simulink model "case4"  (R2024b)
settings: Solver=FixedStepAuto  StartTime=0  StopTime=1  FixedStep=1e-7  RelTol=1e-3
values from neighbouring files (symbols this model uses):
  SG_D_1_D = 0.01056    [IEEE9_case_parameters.m]    (also in case1_parameters.m; case2_parameters.m; case3_parameters.m; case4_parameters.m)
  SG_D_1_EnableSaturation = 0    [IEEE9_case_parameters.m]    (also in case1_parameters.m; case2_parameters.m; case3_parameters.m; case4_parameters.m)
  SG_D_1_f0 = 60    [IEEE9_case_parameters.m]    (also in case1_parameters.m; case2_parameters.m; case3_parameters.m; case4_parameters.m)
  SG_D_1_H = 7.5    [IEEE9_case_parameters.m]    (also in case1_parameters.m; case2_parameters.m; case3_parameters.m; case4_parameters.m)
  SG_D_1_K_A = 20    [IEEE9_case_parameters.m]    (also in case1_parameters.m; case2_parameters.m; case3_parameters.m; case4_parameters.m)
  SG_D_1_K_E = 1.000000e+1    (= 10)    [IEEE9_case_parameters.m]    (also in case1_parameters.m; case2_parameters.m; case3_parameters.m; case4_parameters.m)
  SG_D_1_K_F = 2.363    [IEEE9_case_parameters.m]    (also in case1_parameters.m; case2_parameters.m; case3_parameters.m; case4_parameters.m)
  SG_D_1_K_s = 0.5    [IEEE9_case_parameters.m]    (also in case1_parameters.m = 5; case2_parameters.m = 5; case3_parameters.m = 5; case4_parameters.m = 5)
  SG_D_1_R_a = 0.001088    [IEEE9_case_parameters.m]    (also in case1_parameters.m; case2_parameters.m; case3_parameters.m; case4_parameters.m)
  SG_D_1_S_A = 1    [IEEE9_case_parameters.m]    (also in case1_parameters.m; case2_parameters.m; case3_parameters.m; case4_parameters.m)
  SG_D_1_S_B = 0.103    [IEEE9_case_parameters.m]    (also in case1_parameters.m; case2_parameters.m; case3_parameters.m; case4_parameters.m)
  SG_D_1_S_N = 10.659857    [IEEE9_case_parameters.m]    (also in case1_parameters.m; case2_parameters.m; case3_parameters.m; case4_parameters.m)
  SG_D_1_SpeedPara = 200    [IEEE9_case_parameters.m]    (also in case1_parameters.m; case2_parameters.m; case3_parameters.m; case4_parameters.m)
  SG_D_1_T_0 = 0.720173    [IEEE9_case_parameters.m]    (also in case1_parameters.m = 0.755522; case2_parameters.m = 0.808931; case3_parameters.m = 0.869402; case4_parameters.m = 0.729316)
  SG_D_1_T_1 = 0.3    [IEEE9_case_parameters.m]    (also in case1_parameters.m; case2_parameters.m; case3_parameters.m; case4_parameters.m)
  SG_D_1_T_2 = 0.05    [IEEE9_case_parameters.m]    (also in case1_parameters.m; case2_parameters.m; case3_parameters.m; case4_parameters.m)
  SG_D_1_T_3 = 0.02    [IEEE9_case_parameters.m]    (also in case1_parameters.m; case2_parameters.m; case3_parameters.m; case4_parameters.m)
  SG_D_1_T_4 = 0.005    [IEEE9_case_parameters.m]    (also in case1_parameters.m; case2_parameters.m; case3_parameters.m; case4_parameters.m)
  SG_D_1_T_A = 0.02    [IEEE9_case_parameters.m]    (also in case1_parameters.m; case2_parameters.m; case3_parameters.m; case4_parameters.m)
  SG_D_1_T_dd = 8.000000e+0    (= 8)    [IEEE9_case_parameters.m]    (also in case1_parameters.m; case2_parameters.m; case3_parameters.m; case4_parameters.m)
  SG_D_1_T_ddd = 0.04    [IEEE9_case_parameters.m]    (also in case1_parameters.m; case2_parameters.m; case3_parameters.m; case4_parameters.m)
  SG_D_1_T_E = 0.314    [IEEE9_case_parameters.m]    (also in case1_parameters.m; case2_parameters.m; case3_parameters.m; case4_parameters.m)
  SG_D_1_T_F = 0.35    [IEEE9_case_parameters.m]    (also in case1_parameters.m; case2_parameters.m; case3_parameters.m; case4_parameters.m)
  SG_D_1_T_qd = 0.8    [IEEE9_case_parameters.m]    (also in case1_parameters.m; case2_parameters.m; case3_parameters.m; case4_parameters.m)
  SG_D_1_T_qdd = 0.02    [IEEE9_case_parameters.m]    (also in case1_parameters.m; case2_parameters.m; case3_parameters.m; case4_parameters.m)
  SG_D_1_T_speed = 0.1    [IEEE9_case_parameters.m]    (also in case1_parameters.m = 200; case2_parameters.m = 200; case3_parameters.m = 200; case4_parameters.m = 200)
  SG_D_1_T_w = 0.5    [IEEE9_case_parameters.m]    (also in case1_parameters.m; case2_parameters.m; case3_parameters.m; case4_parameters.m)
  SG_D_1_V_ref = 1.990276    [IEEE9_case_parameters.m]    (also in case1_parameters.m = 2.042296; case2_parameters.m = 2.051388; case3_parameters.m = 2.089584; case4_parameters.m = 2.01845)
  SG_D_1_w_ref = 376.991118    [IEEE9_case_parameters.m]    (also in case1_parameters.m; case2_parameters.m; case3_parameters.m; case4_parameters.m)
  SG_D_1_wb = 6.000000e+1    (= 60)    [IEEE9_case_parameters.m]    (also in case1_parameters.m; case2_parameters.m; case3_parameters.m; case4_parameters.m)
  SG_D_1_x_d = 1.9    [IEEE9_case_parameters.m]    (also in case1_parameters.m; case2_parameters.m; case3_parameters.m; case4_parameters.m)
  SG_D_1_x_dd = 0.302    [IEEE9_case_parameters.m]    (also in case1_parameters.m; case2_parameters.m; case3_parameters.m; case4_parameters.m)
  SG_D_1_x_ddd = 0.204    [IEEE9_case_parameters.m]    (also in case1_parameters.m; case2_parameters.m; case3_parameters.m; case4_parameters.m)
  SG_D_1_x_l = 0.05    [IEEE9_case_parameters.m]    (also in case1_parameters.m; case2_parameters.m; case3_parameters.m; case4_parameters.m)
  SG_D_1_x_q = 1.3    [IEEE9_case_parameters.m]    (also in case1_parameters.m; case2_parameters.m; case3_parameters.m; case4_parameters.m)
  SG_D_1_x_qd = 0.5    [IEEE9_case_parameters.m]    (also in case1_parameters.m; case2_parameters.m; case3_parameters.m; case4_parameters.m)
  SG_D_1_x_qdd = 0.3    [IEEE9_case_parameters.m]    (also in case1_parameters.m; case2_parameters.m; case3_parameters.m; case4_parameters.m)
  SG_D_2_D = 0.02    [IEEE9_case_parameters.m]    (also in case1_parameters.m; case2_parameters.m; case3_parameters.m; case4_parameters.m)
  SG_D_2_EnableSaturation = 0    [IEEE9_case_parameters.m]    (also in case1_parameters.m; case2_parameters.m; case3_parameters.m; case4_parameters.m)
  SG_D_2_f0 = 60    [IEEE9_case_parameters.m]    (also in case1_parameters.m; case2_parameters.m; case3_parameters.m; case4_parameters.m)
  SG_D_2_H = 8.000000e+0    (= 8)    [IEEE9_case_parameters.m]    (also in case1_parameters.m; case2_parameters.m; case3_parameters.m; case4_parameters.m)
  SG_D_2_K_A = 20    [IEEE9_case_parameters.m]    (also in case1_parameters.m; case2_parameters.m; case3_parameters.m; case4_parameters.m)
  SG_D_2_K_E = 1.000000e+1    (= 10)    [IEEE9_case_parameters.m]    (also in case1_parameters.m; case2_parameters.m; case3_parameters.m; case4_parameters.m)
  SG_D_2_K_F = 2.363    [IEEE9_case_parameters.m]    (also in case1_parameters.m; case2_parameters.m; case3_parameters.m; case4_parameters.m)
  SG_D_2_K_s = 0.5    [IEEE9_case_parameters.m]    (also in case1_parameters.m = 4; case2_parameters.m = 4; case3_parameters.m = 4; case4_parameters.m = 4)
  SG_D_2_R_a = 0.001088    [IEEE9_case_parameters.m]    (also in case1_parameters.m; case2_parameters.m; case3_parameters.m; case4_parameters.m)
  SG_D_2_S_A = 1    [IEEE9_case_parameters.m]    (also in case1_parameters.m; case2_parameters.m; case3_parameters.m; case4_parameters.m)
  SG_D_2_S_B = 0.103    [IEEE9_case_parameters.m]    (also in case1_parameters.m; case2_parameters.m; case3_parameters.m; case4_parameters.m)
  SG_D_2_S_N = 10.659857    [IEEE9_case_parameters.m]    (also in case1_parameters.m; case2_parameters.m; case3_parameters.m; case4_parameters.m)
  SG_D_2_SpeedPara = 200    [IEEE9_case_parameters.m]    (also in case1_parameters.m; case2_parameters.m; case3_parameters.m; case4_parameters.m)
  SG_D_2_T_0 = 1.632913    [IEEE9_case_parameters.m]    (also in case1_parameters.m = 1.632925; case2_parameters.m = 1.632915; case3_parameters.m = 1.632914; case4_parameters.m = 1.632927)
  SG_D_2_T_1 = 0.2    [IEEE9_case_parameters.m]    (also in case1_parameters.m; case2_parameters.m; case3_parameters.m; case4_parameters.m)
  SG_D_2_T_2 = 0.05    [IEEE9_case_parameters.m]    (also in case1_parameters.m; case2_parameters.m; case3_parameters.m; case4_parameters.m)
  SG_D_2_T_3 = 0.02    [IEEE9_case_parameters.m]    (also in case1_parameters.m; case2_parameters.m; case3_parameters.m; case4_parameters.m)
  SG_D_2_T_4 = 0.005    [IEEE9_case_parameters.m]    (also in case1_parameters.m; case2_parameters.m; case3_parameters.m; case4_parameters.m)
  SG_D_2_T_A = 0.02    [IEEE9_case_parameters.m]    (also in case1_parameters.m; case2_parameters.m; case3_parameters.m; case4_parameters.m)
  SG_D_2_T_dd = 7.9    [IEEE9_case_parameters.m]    (also in case1_parameters.m; case2_parameters.m; case3_parameters.m; case4_parameters.m)
  SG_D_2_T_ddd = 0.04    [IEEE9_case_parameters.m]    (also in case1_parameters.m; case2_parameters.m; case3_parameters.m; case4_parameters.m)
  SG_D_2_T_E = 0.314    [IEEE9_case_parameters.m]    (also in case1_parameters.m; case2_parameters.m; case3_parameters.m; case4_parameters.m)
  SG_D_2_T_F = 0.35    [IEEE9_case_parameters.m]    (also in case1_parameters.m; case2_parameters.m; case3_parameters.m; case4_parameters.m)
  SG_D_2_T_qd = 0.8    [IEEE9_case_parameters.m]    (also in case1_parameters.m; case2_parameters.m; case3_parameters.m; case4_parameters.m)
  SG_D_2_T_qdd = 0.015    [IEEE9_case_parameters.m]    (also in case1_parameters.m; case2_parameters.m; case3_parameters.m; case4_parameters.m)
  SG_D_2_T_speed = 0.1    [IEEE9_case_parameters.m]    (also in case1_parameters.m = 150; case2_parameters.m = 150; case3_parameters.m = 150; case4_parameters.m = 150)
  SG_D_2_T_w = 0.35    [IEEE9_case_parameters.m]    (also in case1_parameters.m; case2_parameters.m; case3_parameters.m; case4_parameters.m)
  SG_D_2_V_ref = 2.58547    [IEEE9_case_parameters.m]    (also in case1_parameters.m = 2.597896; case2_parameters.m = 2.587136; case3_parameters.m = 2.586042; case4_parameters.m = 2.599679)
  SG_D_2_w_ref = 376.991118    [IEEE9_case_parameters.m]    (also in case1_parameters.m; case2_parameters.m; case3_parameters.m; case4_parameters.m)
  SG_D_2_wb = 6.000000e+1    (= 60)    [IEEE9_case_parameters.m]    (also in case1_parameters.m; case2_parameters.m; case3_parameters.m; case4_parameters.m)
  SG_D_2_x_d = 1.8    [IEEE9_case_parameters.m]    (also in case1_parameters.m; case2_parameters.m; case3_parameters.m; case4_parameters.m)
  SG_D_2_x_dd = 0.302    [IEEE9_case_parameters.m]    (also in case1_parameters.m; case2_parameters.m; case3_parameters.m; case4_parameters.m)
  SG_D_2_x_ddd = 0.204    [IEEE9_case_parameters.m]    (also in case1_parameters.m; case2_parameters.m; case3_parameters.m; case4_parameters.m)
  SG_D_2_x_l = 0.05    [IEEE9_case_parameters.m]    (also in case1_parameters.m; case2_parameters.m; case3_parameters.m; case4_parameters.m)
  SG_D_2_x_q = 1.25    [IEEE9_case_parameters.m]    (also in case1_parameters.m; case2_parameters.m; case3_parameters.m; case4_parameters.m)
  SG_D_2_x_qd = 0.5    [IEEE9_case_parameters.m]    (also in case1_parameters.m; case2_parameters.m; case3_parameters.m; case4_parameters.m)
  SG_D_2_x_qdd = 0.3    [IEEE9_case_parameters.m]    (also in case1_parameters.m; case2_parameters.m; case3_parameters.m; case4_parameters.m)
  SG_D_3_D = 0.02    [IEEE9_case_parameters.m]    (also in case1_parameters.m; case2_parameters.m; case3_parameters.m; case4_parameters.m)
  SG_D_3_EnableSaturation = 0    [IEEE9_case_parameters.m]    (also in case1_parameters.m; case2_parameters.m; case3_parameters.m; case4_parameters.m)
  SG_D_3_f0 = 60    [IEEE9_case_parameters.m]    (also in case1_parameters.m; case2_parameters.m; case3_parameters.m; case4_parameters.m)
  SG_D_3_H = 7.7    [IEEE9_case_parameters.m]    (also in case1_parameters.m; case2_parameters.m; case3_parameters.m; case4_parameters.m)
  SG_D_3_K_A = 20    [IEEE9_case_parameters.m]    (also in case1_parameters.m; case2_parameters.m; case3_parameters.m; case4_parameters.m)
  SG_D_3_K_E = 1.000000e+1    (= 10)    [IEEE9_case_parameters.m]    (also in case1_parameters.m; case2_parameters.m; case3_parameters.m; case4_parameters.m)
  SG_D_3_K_F = 2.363    [IEEE9_case_parameters.m]    (also in case1_parameters.m; case2_parameters.m; case3_parameters.m; case4_parameters.m)
  SG_D_3_K_s = 0.2    [IEEE9_case_parameters.m]    (also in case1_parameters.m = 2; case2_parameters.m = 2; case3_parameters.m = 2; case4_parameters.m = 2)
  SG_D_3_R_a = 0.001088    [IEEE9_case_parameters.m]    (also in case1_parameters.m; case2_parameters.m; case3_parameters.m; case4_parameters.m)
  SG_D_3_S_A = 1    [IEEE9_case_parameters.m]    (also in case1_parameters.m; case2_parameters.m; case3_parameters.m; case4_parameters.m)
  SG_D_3_S_B = 0.103    [IEEE9_case_parameters.m]    (also in case1_parameters.m; case2_parameters.m; case3_parameters.m; case4_parameters.m)
  SG_D_3_S_N = 10.659857    [IEEE9_case_parameters.m]    (also in case1_parameters.m; case2_parameters.m; case3_parameters.m; case4_parameters.m)
  SG_D_3_SpeedPara = 200    [IEEE9_case_parameters.m]    (also in case1_parameters.m; case2_parameters.m; case3_parameters.m; case4_parameters.m)
  SG_D_3_T_0 = 0.850788    [IEEE9_case_parameters.m]    (also in case1_parameters.m = 0.850786; case2_parameters.m = 0.850787; case3_parameters.m; case4_parameters.m = 0.850786)
  SG_D_3_T_1 = 0.2    [IEEE9_case_parameters.m]    (also in case1_parameters.m; case2_parameters.m; case3_parameters.m; case4_parameters.m)
  SG_D_3_T_2 = 0.05    [IEEE9_case_parameters.m]    (also in case1_parameters.m; case2_parameters.m; case3_parameters.m; case4_parameters.m)
  SG_D_3_T_3 = 0.02    [IEEE9_case_parameters.m]    (also in case1_parameters.m; case2_parameters.m; case3_parameters.m; case4_parameters.m)
  SG_D_3_T_4 = 0.005    [IEEE9_case_parameters.m]    (also in case1_parameters.m; case2_parameters.m; case3_parameters.m; case4_parameters.m)
  SG_D_3_T_A = 0.02    [IEEE9_case_parameters.m]    (also in case1_parameters.m; case2_parameters.m; case3_parameters.m; case4_parameters.m)
  SG_D_3_T_dd = 8.1    [IEEE9_case_parameters.m]    (also in case1_parameters.m; case2_parameters.m; case3_parameters.m; case4_parameters.m)
  SG_D_3_T_ddd = 0.04    [IEEE9_case_parameters.m]    (also in case1_parameters.m; case2_parameters.m; case3_parameters.m; case4_parameters.m)
  SG_D_3_T_E = 0.314    [IEEE9_case_parameters.m]    (also in case1_parameters.m; case2_parameters.m; case3_parameters.m; case4_parameters.m)
  SG_D_3_T_F = 0.35    [IEEE9_case_parameters.m]    (also in case1_parameters.m; case2_parameters.m; case3_parameters.m; case4_parameters.m)
  SG_D_3_T_qd = 0.8    [IEEE9_case_parameters.m]    (also in case1_parameters.m; case2_parameters.m; case3_parameters.m; case4_parameters.m)
  SG_D_3_T_qdd = 0.015    [IEEE9_case_parameters.m]    (also in case1_parameters.m; case2_parameters.m; case3_parameters.m; case4_parameters.m)
  SG_D_3_T_speed = 0.1    [IEEE9_case_parameters.m]    (also in case1_parameters.m = 180; case2_parameters.m = 180; case3_parameters.m = 180; case4_parameters.m = 180)
  SG_D_3_T_w = 0.4    [IEEE9_case_parameters.m]    (also in case1_parameters.m; case2_parameters.m; case3_parameters.m; case4_parameters.m)
  SG_D_3_V_ref = 1.892727    [IEEE9_case_parameters.m]    (also in case1_parameters.m = 1.906439; case2_parameters.m = 1.895535; case3_parameters.m = 1.892105; case4_parameters.m = 1.906598)
  SG_D_3_w_ref = 376.991118    [IEEE9_case_parameters.m]    (also in case1_parameters.m; case2_parameters.m; case3_parameters.m; case4_parameters.m)
  SG_D_3_wb = 6.000000e+1    (= 60)    [IEEE9_case_parameters.m]    (also in case1_parameters.m; case2_parameters.m; case3_parameters.m; case4_parameters.m)
  SG_D_3_x_d = 1.85    [IEEE9_case_parameters.m]    (also in case1_parameters.m; case2_parameters.m; case3_parameters.m; case4_parameters.m)
  SG_D_3_x_dd = 0.302    [IEEE9_case_parameters.m]    (also in case1_parameters.m; case2_parameters.m; case3_parameters.m; case4_parameters.m)
  SG_D_3_x_ddd = 0.204    [IEEE9_case_parameters.m]    (also in case1_parameters.m; case2_parameters.m; case3_parameters.m; case4_parameters.m)
  SG_D_3_x_l = 0.05    [IEEE9_case_parameters.m]    (also in case1_parameters.m; case2_parameters.m; case3_parameters.m; case4_parameters.m)
  SG_D_3_x_q = 1.2    [IEEE9_case_parameters.m]    (also in case1_parameters.m; case2_parameters.m; case3_parameters.m; case4_parameters.m)
  SG_D_3_x_qd = 0.5    [IEEE9_case_parameters.m]    (also in case1_parameters.m; case2_parameters.m; case3_parameters.m; case4_parameters.m)
  SG_D_3_x_qdd = 0.3    [IEEE9_case_parameters.m]    (also in case1_parameters.m; case2_parameters.m; case3_parameters.m; case4_parameters.m)
(part 7 of 12)

== system case4/SG_D_2/T_e_SG_D_2_block ==
  note: T_e_SG_D_2 in case4
      | $-\frac{\psi _{d,\mathrm{SG},D,2}\,\left(\psi _{q,\mathrm{SG},D,2}+\frac{\psi _{\mathrm{gq},\mathrm{SG},D,2}\,\left(x_{l}-x_{\mathrm{qdd}}\right)}{x_{l}-x_{\mathrm{qd}}}+\frac{\psi _{\mathrm{kq},\mathrm{SG},D,2}\,\left(x_{\mathrm{qd}}-x_{\mathrm{qdd}}\right)}{x_{l}-x_{\mathrm{qd}}}\right)}{x_{\mathrm{qdd}}}-\frac{\psi _{q,\mathrm{SG},D,2}\,\left(\frac{\psi _{\mathrm{1d},\mathrm{SG},D,2}\,\left(x_{\mathrm{dd}}-x_{\mathrm{ddd}}\right)}{x_{\mathrm{dd}}-x_{l}}-\psi _{d,\mathrm{SG},D,2}+\frac{\psi _{\mathrm{fd},\mathrm{SG},D,2}\,\left(x_{\mathrm{ddd}}-x_{l}\right)}{x_{\mathrm{dd}}-x_{l}}\right)}{x_{\mathrm{ddd}}}$
      | Automatically generated on 2025-10-31 19:06:05 .
  State_psi_d_SG_D_2_11756 : Inport
  State_psi_gq_SG_D_2_3103f : Inport  Port=2
  State_psi_kq_SG_D_2_da24b : Inport  Port=3
  State_psi_q_SG_D_2_38137 : Inport  Port=4
  State_psi_q_SG_D_2_ed317 : Inport  Port=5
  State_psi_1d_SG_D_2_6920c : Inport  Port=6
  State_psi_d_SG_D_2_9e42d : Inport  Port=7
  State_psi_fd_SG_D_2_0e9d9 : Inport  Port=8
  Add_2c7a9 : Sum
  Add_44fa7 : Sum
  Add_47e7d : Sum
  Add_73c7b : Sum
  Add_b7626 : Sum
  Add_b8887 : Sum
  Constant_-1_0949c : Constant  Value=-1
  Constant_-1_0dd71 : Constant  Value=-1
  Constant_-1_7cacd : Constant  Value=-1
  Constant_-1_ce45c : Constant  Value=-1
  Constant_-1_f8543 : Constant  Value=-1
  Constant_x_dd_66c3f : Constant  Value=x_dd
  Constant_x_dd_9b39c : Constant  Value=x_dd
  Constant_x_dd_ec85b : Constant  Value=x_dd
  Constant_x_ddd_e09db : Constant  Value=x_ddd
  Constant_x_ddd_e945b : Constant  Value=x_ddd
  Constant_x_ddd_f556b : Constant  Value=x_ddd
  Constant_x_l_46472 : Constant  Value=x_l
  Constant_x_l_7373e : Constant  Value=x_l
  Constant_x_l_77990 : Constant  Value=x_l
  Constant_x_l_874fd : Constant  Value=x_l
  Constant_x_l_ca8fe : Constant  Value=x_l
  Constant_x_l_d87e3 : Constant  Value=x_l
  Constant_x_qd_2f18d : Constant  Value=x_qd
  Constant_x_qd_31197 : Constant  Value=x_qd
  Constant_x_qd_3fd95 : Constant  Value=x_qd
  Constant_x_qdd_6d3e7 : Constant  Value=x_qdd
  Constant_x_qdd_aa4a8 : Constant  Value=x_qdd
  Constant_x_qdd_ddfb4 : Constant  Value=x_qdd
  Divide_10c09 : Product  Inputs=*/
  Divide_125e8 : Product  Inputs=*/
  Divide_291f1 : Product  Inputs=*/
  Divide_59e24 : Product  Inputs=*/
  Divide_6386a : Product  Inputs=*/
  Divide_88896 : Product  Inputs=*/
  Product_127af : Product
  Product_16d66 : Product
  Product_5984f : Product
  Product_70f67 : Product
  Product_766ec : Product
  Product_94b3f : Product
  Product_b0cc7 : Product
  Product_dd356 : Product
  Product_e4c88 : Product
  Product_e618a : Product
  Product_f1edd : Product
  Subtract_24c52 : Sum  Inputs=+-
  Subtract_2830b : Sum  Inputs=+-
  Subtract_4a8ab : Sum  Inputs=+-
  Subtract_8aa99 : Sum  Inputs=+-
  Subtract_a0ad2 : Sum  Inputs=+-
  Subtract_a7382 : Sum  Inputs=+-
  Subtract_bad0d : Sum  Inputs=+-
  Blockout_T_e_SG_D_2_aeb34 : Outport
  wires:
  Constant_-1_7cacd/1 -> Product_94b3f/1
  Divide_291f1/1 -> Subtract_2830b/1
  Constant_-1_f8543/1 -> Product_b0cc7/1
  Constant_x_l_7373e/1 -> Product_b0cc7/2
  Constant_x_qd_31197/1 -> Subtract_a0ad2/1
  Product_16d66/1 -> Divide_291f1/1
  Product_b0cc7/1 -> Add_b7626/1
  Divide_6386a/1 -> Subtract_24c52/2
  Constant_x_qdd_ddfb4/1 -> Subtract_a0ad2/2
  Constant_x_qdd_6d3e7/1 -> Divide_10c09/2
  Constant_x_ddd_e09db/1 -> Subtract_a7382/2
  Constant_x_qdd_aa4a8/1 -> Add_b7626/2
  Constant_x_l_874fd/1 -> Product_94b3f/2
  Constant_-1_0dd71/1 -> Product_127af/1
  Constant_x_l_d87e3/1 -> Product_127af/2
  Constant_-1_0949c/1 -> Product_766ec/1
  State_psi_1d_SG_D_2_6920c/1 -> Product_766ec/2
  Constant_x_dd_66c3f/1 -> Subtract_a7382/1
  Divide_88896/1 -> Subtract_2830b/2
  State_psi_gq_SG_D_2_3103f/1 -> Product_16d66/1
  Add_b7626/1 -> Product_16d66/2
  Subtract_2830b/1 -> Add_44fa7/1
  Constant_x_dd_ec85b/1 -> Subtract_bad0d/1
  Product_94b3f/1 -> Add_47e7d/1
  Product_e618a/1 -> Product_e4c88/1
  Constant_x_qd_2f18d/1 -> Add_47e7d/2
  State_psi_kq_SG_D_2_da24b/1 -> Product_70f67/1
  Subtract_a0ad2/1 -> Product_70f67/2
  Product_127af/1 -> Add_2c7a9/1
  State_psi_q_SG_D_2_ed317/1 -> Product_dd356/1
  Constant_x_qd_3fd95/1 -> Add_2c7a9/2
  Product_766ec/1 -> Product_f1edd/1
  Divide_125e8/1 -> Add_b8887/2
  Subtract_a7382/1 -> Product_f1edd/2
  Constant_x_l_46472/1 -> Subtract_bad0d/2
  Constant_x_ddd_f556b/1 -> Subtract_4a8ab/1
  Constant_x_dd_9b39c/1 -> Subtract_8aa99/1
  Constant_x_l_ca8fe/1 -> Subtract_4a8ab/2
  Add_b8887/1 -> Blockout_T_e_SG_D_2_aeb34/1
  Add_47e7d/1 -> Divide_291f1/2
  Product_70f67/1 -> Divide_88896/1
  Product_e4c88/1 -> Divide_10c09/1
  State_psi_d_SG_D_2_11756/1 -> Product_e618a/2
  Add_2c7a9/1 -> Divide_88896/2
  Product_f1edd/1 -> Divide_59e24/1
  Subtract_bad0d/1 -> Divide_59e24/2
  Constant_x_l_77990/1 -> Subtract_8aa99/2
  State_psi_fd_SG_D_2_0e9d9/1 -> Product_5984f/1
  Constant_x_ddd_e945b/1 -> Divide_125e8/2
  Product_dd356/1 -> Divide_125e8/1
  Subtract_4a8ab/1 -> Product_5984f/2
  Divide_59e24/1 -> Add_73c7b/1
  State_psi_d_SG_D_2_9e42d/1 -> Add_73c7b/2
  Add_73c7b/1 -> Subtract_24c52/1
  Product_5984f/1 -> Divide_6386a/1
  Subtract_8aa99/1 -> Divide_6386a/2
  Constant_-1_ce45c/1 -> Product_e618a/1
  State_psi_q_SG_D_2_38137/1 -> Add_44fa7/2
  Add_44fa7/1 -> Product_e4c88/2
  Subtract_24c52/1 -> Product_dd356/2
  Divide_10c09/1 -> Add_b8887/1

== system case4/SG_D_2/d_E_fd_SG_D_2_block ==
  note: d_E_fd_SG_D_2 in case4
      | $\frac{V_{f,\mathrm{SG},D,2}-E_{\mathrm{fd},\mathrm{SG},D,2}\,K_{E}}{T_{E}}$
      | Automatically generated on 2025-10-31 19:05:49 .
  State_E_fd_SG_D_2_90b3d : Inport
  State_V_f_SG_D_2_8bae1 : Inport  Port=2
  Add_95d66 : Sum
  Constant_-1_0fe84 : Constant  Value=-1
  Constant_K_E_f5d65 : Constant  Value=K_E
  Constant_T_E_c64ad : Constant  Value=T_E
  Divide_72050 : Product  Inputs=*/
  Product_4c4c6 : Product
  Product_de249 : Product
  Blockout_d_E_fd_SG_D_2_ce12b : Outport
  wires:
  Constant_-1_0fe84/1 -> Product_4c4c6/1
  State_E_fd_SG_D_2_90b3d/1 -> Product_4c4c6/2
  Product_4c4c6/1 -> Product_de249/1
  Constant_K_E_f5d65/1 -> Product_de249/2
  Product_de249/1 -> Add_95d66/1
  Constant_T_E_c64ad/1 -> Divide_72050/2
  State_V_f_SG_D_2_8bae1/1 -> Add_95d66/2
  Add_95d66/1 -> Divide_72050/1
  Divide_72050/1 -> Blockout_d_E_fd_SG_D_2_ce12b/1

== system case4/SG_D_2/d_Px_1_SG_D_2_block ==
  note: d_Px_1_SG_D_2 in case4
      | $\frac{w_{\mathrm{SG},D,2}-2\,\pi \,f_{0}}{T_{w}}-\frac{\mathrm{Px}_{1,\mathrm{SG},D,2}}{T_{w}}$
      | Automatically generated on 2025-10-31 19:05:50 .
  State_Px_1_SG_D_2_ffc5d : Inport
  State_w_SG_D_2_89096 : Inport  Port=2
  Add_5c420 : Sum
  Add_9f309 : Sum
  Constant_-1_27984 : Constant  Value=-1
  Constant_-2.0_1968b : Constant  Value=-2.0
  Constant_T_w_6d8bf : Constant  Value=T_w
  Constant_T_w_fd983 : Constant  Value=T_w
  Constant_f0_3c00a : Constant  Value=f0
  Constant_pi_a557c : Constant  Value=pi
  Divide_17f61 : Product  Inputs=*/
  Divide_d9b7f : Product  Inputs=*/
  Product_78a16 : Product
  Product_83968 : Product
  Product_8d6e2 : Product
  Blockout_d_Px_1_SG_D_2_f7300 : Outport
  wires:
  Constant_-2.0_1968b/1 -> Product_83968/1
  State_w_SG_D_2_89096/1 -> Add_9f309/2
  Constant_pi_a557c/1 -> Product_83968/2
  Product_83968/1 -> Product_78a16/1
  Constant_f0_3c00a/1 -> Product_78a16/2
  Constant_-1_27984/1 -> Product_8d6e2/1
  State_Px_1_SG_D_2_ffc5d/1 -> Product_8d6e2/2
  Product_78a16/1 -> Add_9f309/1
  Product_8d6e2/1 -> Divide_17f61/1
  Constant_T_w_6d8bf/1 -> Divide_17f61/2
  Add_9f309/1 -> Divide_d9b7f/1
  Constant_T_w_fd983/1 -> Divide_d9b7f/2
  Divide_17f61/1 -> Add_5c420/1
  Divide_d9b7f/1 -> Add_5c420/2
  Add_5c420/1 -> Blockout_d_Px_1_SG_D_2_f7300/1

== system case4/SG_D_2/d_Px_2_SG_D_2_block ==
  note: d_Px_2_SG_D_2 in case4
      | $\frac{\mathrm{Px}_{1,\mathrm{SG},D,2}-T_{2}\,\left(\frac{\mathrm{Px}_{1,\mathrm{SG},D,2}}{T_{w}}-\frac{w_{\mathrm{SG},D,2}-2\,\pi \,f_{0}}{T_{w}}\right)}{T_{1}}-\frac{\mathrm{Px}_{2,\mathrm{SG},D,2}}{T_{1}}$
      | Automatically generated on 2025-10-31 19:05:51 .
  State_Px_2_SG_D_2_0c5e7 : Inport
  State_Px_1_SG_D_2_d066c : Inport  Port=2
  State_Px_1_SG_D_2_9542b : Inport  Port=3
  State_w_SG_D_2_251c8 : Inport  Port=4
  Add_54564 : Sum
  Add_5d193 : Sum
  Add_b89c3 : Sum
  Add_bfc67 : Sum
  Constant_-1_3d68c : Constant  Value=-1
  Constant_-1_b7b4c : Constant  Value=-1
  Constant_-2.0_a3c7b : Constant  Value=-2.0
  Constant_T_1_c2f5d : Constant  Value=T_1
  Constant_T_1_df662 : Constant  Value=T_1
  Constant_T_2_79b79 : Constant  Value=T_2
  Constant_T_w_40fdc : Constant  Value=T_w
  Constant_T_w_4ad23 : Constant  Value=T_w
  Constant_f0_56b41 : Constant  Value=f0
  Constant_pi_103cb : Constant  Value=pi
  Divide_1ad7b : Product  Inputs=*/
  Divide_1f7ab : Product  Inputs=*/
  Divide_27c9e : Product  Inputs=*/
  Divide_96b21 : Product  Inputs=*/
  Product_09bcf : Product
  Product_54d9a : Product
  Product_5f47b : Product
  Product_62beb : Product
  Product_cd1c0 : Product
  Blockout_d_Px_2_SG_D_2_a31a2 : Outport
  wires:
  Constant_-1_b7b4c/1 -> Product_54d9a/1
  Constant_-2.0_a3c7b/1 -> Product_5f47b/1
  Product_09bcf/1 -> Add_bfc67/2
  State_w_SG_D_2_251c8/1 -> Add_b89c3/2
  Constant_pi_103cb/1 -> Product_5f47b/2
  Product_5f47b/1 -> Product_cd1c0/1
  State_Px_1_SG_D_2_9542b/1 -> Product_62beb/2
  Constant_f0_56b41/1 -> Product_cd1c0/2
  State_Px_2_SG_D_2_0c5e7/1 -> Product_54d9a/2
  Constant_-1_3d68c/1 -> Product_62beb/1
  Product_cd1c0/1 -> Add_b89c3/1
  Product_62beb/1 -> Divide_1f7ab/1
  Constant_T_w_40fdc/1 -> Divide_1f7ab/2
  Add_b89c3/1 -> Divide_96b21/1
  Constant_T_w_4ad23/1 -> Divide_96b21/2
  Divide_1f7ab/1 -> Add_54564/1
  Divide_96b21/1 -> Add_54564/2
  Constant_T_2_79b79/1 -> Product_09bcf/1
  Add_54564/1 -> Product_09bcf/2
  State_Px_1_SG_D_2_d066c/1 -> Add_bfc67/1
  Product_54d9a/1 -> Divide_27c9e/1
  Constant_T_1_df662/1 -> Divide_27c9e/2
  Add_bfc67/1 -> Divide_1ad7b/1
  Constant_T_1_c2f5d/1 -> Divide_1ad7b/2
  Divide_27c9e/1 -> Add_5d193/1
  Divide_1ad7b/1 -> Add_5d193/2
  Add_5d193/1 -> Blockout_d_Px_2_SG_D_2_a31a2/1

== system case4/SG_D_2/d_Px_3_SG_D_2_block ==
  note: d_Px_3_SG_D_2 in case4
      | $\frac{\mathrm{Px}_{2,\mathrm{SG},D,2}+T_{4}\,\left(\frac{\mathrm{Px}_{1,\mathrm{SG},D,2}-T_{2}\,\left(\frac{\mathrm{Px}_{1,\mathrm{SG},D,2}}{T_{w}}-\frac{w_{\mathrm{SG},D,2}-2\,\pi \,f_{0}}{T_{w}}\right)}{T_{1}}-\frac{\mathrm{Px}_{2,\mathrm{SG},D,2}}{T_{1}}\right)}{T_{3}}-\frac{\mathrm{Px}_{3,\mathrm{SG},D,2}}{T_{3}}$
      | Automatically generated on 2025-10-31 19:05:54 .
  State_Px_3_SG_D_2_1b144 : Inport
  State_Px_2_SG_D_2_117c1 : Inport  Port=2
  State_Px_2_SG_D_2_e0625 : Inport  Port=3
  State_Px_1_SG_D_2_71ec3 : Inport  Port=4
  State_Px_1_SG_D_2_7e22a : Inport  Port=5
  State_w_SG_D_2_cceda : Inport  Port=6
  Add_08121 : Sum
  Add_4736c : Sum
  Add_548e3 : Sum
  Add_69d12 : Sum
  Add_9221e : Sum
  Add_f82c5 : Sum
  Constant_-1_0714c : Constant  Value=-1
  Constant_-1_0bf0f : Constant  Value=-1
  Constant_-1_5d4d6 : Constant  Value=-1
  Constant_-2.0_f2798 : Constant  Value=-2.0
  Constant_T_1_45d10 : Constant  Value=T_1
  Constant_T_1_b70a7 : Constant  Value=T_1
  Constant_T_2_ac8f1 : Constant  Value=T_2
  Constant_T_3_03ac1 : Constant  Value=T_3
  Constant_T_3_454e9 : Constant  Value=T_3
  Constant_T_4_05f3b : Constant  Value=T_4
  Constant_T_w_487c9 : Constant  Value=T_w
  Constant_T_w_bc33d : Constant  Value=T_w
  Constant_f0_9da41 : Constant  Value=f0
  Constant_pi_88d9b : Constant  Value=pi
  Divide_3d3cf : Product  Inputs=*/
  Divide_556f3 : Product  Inputs=*/
  Divide_9fca9 : Product  Inputs=*/
  Divide_b1640 : Product  Inputs=*/
  Divide_bb34a : Product  Inputs=*/
  Divide_bc21c : Product  Inputs=*/
  Product_64562 : Product
  Product_68fcf : Product
  Product_a71bf : Product
  Product_cb2a5 : Product
  Product_da8a1 : Product
  Product_eae51 : Product
  Product_fc825 : Product
  Blockout_d_Px_3_SG_D_2_a07c3 : Outport
  wires:
  Constant_-2.0_f2798/1 -> Product_a71bf/1
  State_w_SG_D_2_cceda/1 -> Add_4736c/2
  Add_69d12/1 -> Divide_9fca9/1
  Constant_pi_88d9b/1 -> Product_a71bf/2
  Constant_-1_0714c/1 -> Product_64562/1
  Product_a71bf/1 -> Product_68fcf/1
  State_Px_2_SG_D_2_e0625/1 -> Product_64562/2
  State_Px_1_SG_D_2_7e22a/1 -> Product_da8a1/2
  Divide_9fca9/1 -> Add_f82c5/2
  Constant_f0_9da41/1 -> Product_68fcf/2
  Constant_-1_0bf0f/1 -> Product_da8a1/1
  Product_68fcf/1 -> Add_4736c/1
  Product_da8a1/1 -> Divide_bc21c/1
  Constant_T_w_487c9/1 -> Divide_bc21c/2
  Divide_b1640/1 -> Add_f82c5/1
  Add_4736c/1 -> Divide_556f3/1
  Product_eae51/1 -> Add_548e3/2
  Constant_T_w_bc33d/1 -> Divide_556f3/2
  Divide_bc21c/1 -> Add_08121/1
  State_Px_1_SG_D_2_71ec3/1 -> Add_548e3/1
  Divide_556f3/1 -> Add_08121/2
  Constant_-1_5d4d6/1 -> Product_cb2a5/1
  Constant_T_2_ac8f1/1 -> Product_eae51/1
  Add_08121/1 -> Product_eae51/2
  Product_64562/1 -> Divide_3d3cf/1
  Constant_T_1_b70a7/1 -> Divide_3d3cf/2
  Add_548e3/1 -> Divide_bb34a/1
  Constant_T_1_45d10/1 -> Divide_bb34a/2
  Divide_3d3cf/1 -> Add_9221e/1
  Divide_bb34a/1 -> Add_9221e/2
  Constant_T_4_05f3b/1 -> Product_fc825/1
  Add_9221e/1 -> Product_fc825/2
  State_Px_3_SG_D_2_1b144/1 -> Product_cb2a5/2
  State_Px_2_SG_D_2_117c1/1 -> Add_69d12/1
  Product_fc825/1 -> Add_69d12/2
  Product_cb2a5/1 -> Divide_b1640/1
  Constant_T_3_454e9/1 -> Divide_b1640/2
  Constant_T_3_03ac1/1 -> Divide_9fca9/2
  Add_f82c5/1 -> Blockout_d_Px_3_SG_D_2_a07c3/1

== system case4/SG_D_2/d_R_f_SG_D_2_block ==
  note: d_R_f_SG_D_2 in case4
      | $-\frac{R_{f,\mathrm{SG},D,2}-\frac{E_{\mathrm{fd},\mathrm{SG},D,2}\,K_{F}}{T_{F}}}{T_{F}}$
      | Automatically generated on 2025-10-31 19:05:48 .
  State_E_fd_SG_D_2_6574e : Inport
  State_R_f_SG_D_2_f9839 : Inport  Port=2
  Constant_K_F_9b2d2 : Constant  Value=K_F
  Constant_T_F_8de8b : Constant  Value=T_F
  Constant_T_F_fc57e : Constant  Value=T_F
  Divide_1921e : Product  Inputs=*/
  Divide_6734f : Product  Inputs=*/
  Product_c3d09 : Product
  Subtract_ea807 : Sum  Inputs=+-
  Blockout_d_R_f_SG_D_2_5255c : Outport
  wires:
  Constant_T_F_fc57e/1 -> Divide_6734f/2
  State_E_fd_SG_D_2_6574e/1 -> Product_c3d09/1
  Constant_K_F_9b2d2/1 -> Product_c3d09/2
  State_R_f_SG_D_2_f9839/1 -> Subtract_ea807/2
  Product_c3d09/1 -> Divide_6734f/1
  Divide_6734f/1 -> Subtract_ea807/1
  Constant_T_F_8de8b/1 -> Divide_1921e/2
  Subtract_ea807/1 -> Divide_1921e/1
  Divide_1921e/1 -> Blockout_d_R_f_SG_D_2_5255c/1

== system case4/SG_D_2/d_T_m_SG_D_2_block ==
  note: d_T_m_SG_D_2 in case4
      | $-\frac{T_{m,\mathrm{SG},D,2}-T_{0}+\frac{\mathrm{SpeedPara}\,\left(w_{\mathrm{SG},D,2}-w_{\mathrm{ref}}\right)}{2\,f_{0}\,\pi }}{T_{\mathrm{speed}}}$
      | Automatically generated on 2025-10-31 19:05:40 .
  State_w_SG_D_2_20fb2 : Inport
  State_T_m_SG_D_2_247d7 : Inport  Port=2
  Add_bb900 : Sum
  Add_be9d5 : Sum
  Constant_-1_af39f : Constant  Value=-1
  Constant_2.0_4ffad : Constant  Value=2.0
  Constant_SpeedPara_5074d : Constant  Value=SpeedPara
  Constant_T_0_1ef5a : Constant  Value=T_0
  Constant_T_speed_897f7 : Constant  Value=T_speed
  Constant_f0_08270 : Constant  Value=f0
  Constant_pi_2460d : Constant  Value=pi
  Constant_w_ref_f3fa2 : Constant  Value=w_ref
  Divide_79857 : Product  Inputs=*/
  Divide_905b4 : Product  Inputs=*/
  Product_62488 : Product
  Product_c28b9 : Product
  Product_c30b0 : Product
  Product_ec04a : Product
  Subtract_d7440 : Sum  Inputs=+-
  Blockout_d_T_m_SG_D_2_16fb0 : Outport
  wires:
  Constant_pi_2460d/1 -> Product_62488/2
  Constant_-1_af39f/1 -> Product_c28b9/1
  Constant_w_ref_f3fa2/1 -> Add_be9d5/2
  State_w_SG_D_2_20fb2/1 -> Product_c28b9/2
  Product_c28b9/1 -> Add_be9d5/1
  Add_bb900/1 -> Subtract_d7440/1
  Add_be9d5/1 -> Product_ec04a/2
  Constant_2.0_4ffad/1 -> Product_62488/1
  Constant_SpeedPara_5074d/1 -> Product_ec04a/1
  Product_62488/1 -> Product_c30b0/1
  Constant_f0_08270/1 -> Product_c30b0/2
  Product_ec04a/1 -> Divide_79857/1
  Product_c30b0/1 -> Divide_79857/2
  Divide_79857/1 -> Add_bb900/1
  Constant_T_0_1ef5a/1 -> Add_bb900/2
  State_T_m_SG_D_2_247d7/1 -> Subtract_d7440/2
  Subtract_d7440/1 -> Divide_905b4/1
  Constant_T_speed_897f7/1 -> Divide_905b4/2
  Divide_905b4/1 -> Blockout_d_T_m_SG_D_2_16fb0/1

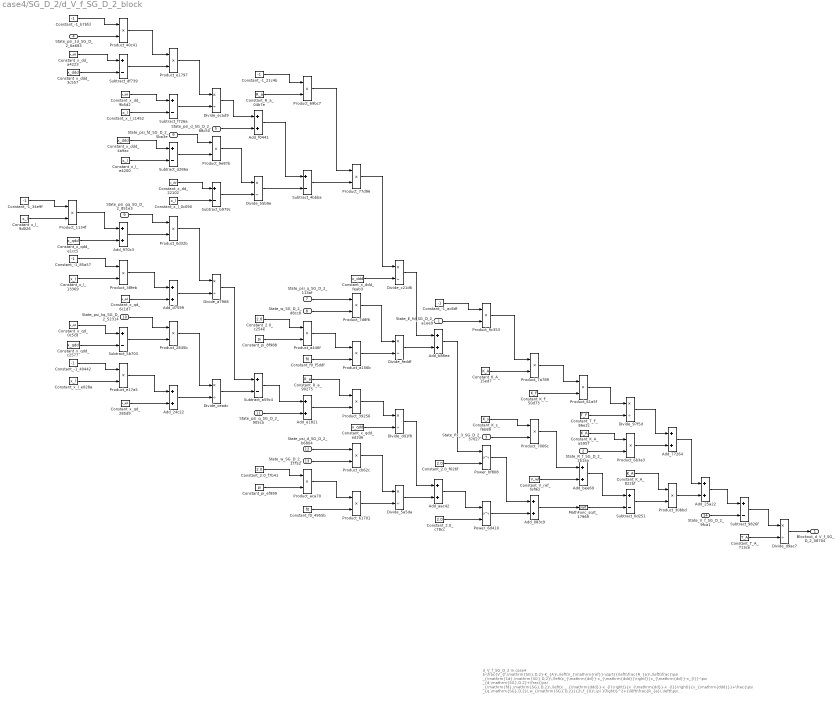
== system case4/SG_D_2/d_V_f_SG_D_2_block ==
  note: d_V_f_SG_D_2 in case4
      | $-\frac{V_{f,\mathrm{SG},D,2}-K_{A}\,\left(V_{\mathrm{ref}}-\sqrt{{\left(\frac{R_{a}\,\left(\frac{\psi _{\mathrm{1d},\mathrm{SG},D,2}\,\left(x_{\mathrm{dd}}-x_{\mathrm{ddd}}\right)}{x_{\mathrm{dd}}-x_{l}}-\psi _{d,\mathrm{SG},D,2}+\frac{\psi _{\mathrm{fd},\mathrm{SG},D,2}\,\left(x_{\mathrm{ddd}}-x_{l}\right)}{x_{\mathrm{dd}}-x_{l}}\right)}{x_{\mathrm{ddd}}}+\frac{\psi _{q,\mathrm{SG},D,2}\,w_{\mathrm{SG},D,2}}{2\,f_{0}\,\pi }\right)}^2+{\left(\frac{R_{a}\,\left(\psi _{q,\mathrm{SG},D,2}+\frac{\psi _{\mathrm{gq},\mathrm{SG},D,2}\,\left(x_{l}-x_{\mathrm{qdd}}\right)}{x_{l}-x_{\mathrm{qd}}}+\frac{\psi _{\mathrm{kq},\mathrm{SG},D,2}\,\left(x_{\mathrm{qd}}-x_{\mathrm{qdd}}\right)}{x_{l}-x_{\mathrm{qd}}}\right)}{x_{\mathrm{qdd}}}+\frac{\psi _{d,\mathrm{SG},D,2}\,w_{\mathrm{SG},D,2}}{2\,f_{0}\,\pi }\right)}^2}+K_{s}\,\mathrm{Px}_{3,\mathrm{SG},D,2}\right)-K_{A}\,R_{f,\mathrm{SG},D,2}+\frac{E_{\mathrm{fd},\mathrm{SG},D,2}\,K_{A}\,K_{F}}{T_{F}}}{T_{A}}$
      | Automatically generated on 2025-10-31 19:05:47 .
  State_E_fd_SG_D_2_a1ee9 : Inport
  State_R_f_SG_D_2_2b1aa : Inport  Port=2
  State_Px_3_SG_D_2_37027 : Inport  Port=3
  State_psi_1d_SG_D_2_6a683 : Inport  Port=4
  State_psi_d_SG_D_2_88c50 : Inport  Port=5
  State_psi_fd_SG_D_2_5ba3e : Inport  Port=6
  State_psi_q_SG_D_2_113af : Inport  Port=7
  State_w_SG_D_2_d8cc8 : Inport  Port=8
  State_psi_gq_SG_D_2_851e3 : Inport  Port=9
  State_psi_kq_SG_D_2_52314 : Inport  Port=10
  State_psi_q_SG_D_2_905ca : Inport  Port=11
  State_psi_d_SG_D_2_b6804 : Inport  Port=12
  State_w_SG_D_2_1f752 : Inport  Port=13
  State_V_f_SG_D_2_9fca1 : Inport  Port=14
  Add_083c9 : Sum
  Add_24c22 : Sum
  Add_25a22 : Sum
  Add_77264 : Sum
  Add_970c3 : Sum
  Add_aac42 : Sum
  Add_b86ea : Sum
  Add_bee69 : Sum
  Add_d7599 : Sum
  Add_e1821 : Sum
  Add_f0441 : Sum
  Constant_-1_21c4b : Constant  Value=-1
  Constant_-1_34e9f : Constant  Value=-1
  Constant_-1_40442 : Constant  Value=-1
  Constant_-1_85a57 : Constant  Value=-1
  Constant_-1_ac8df : Constant  Value=-1
  Constant_-1_b7bfd : Constant  Value=-1
  Constant_2.0_c254e : Constant  Value=2.0
  Constant_2.0_c78cc : Constant  Value=2.0
  Constant_2.0_f026f : Constant  Value=2.0
  Constant_2.0_f7b41 : Constant  Value=2.0
  Constant_K_A_15ed7 : Constant  Value=K_A
  Constant_K_A_822bf : Constant  Value=K_A
  Constant_K_A_a5957 : Constant  Value=K_A
  Constant_K_F_50d73 : Constant  Value=K_F
  Constant_K_s_f6b89 : Constant  Value=K_s
  Constant_R_a_04b7e : Constant  Value=R_a
  Constant_R_a_90275 : Constant  Value=R_a
  Constant_T_A_713ce : Constant  Value=T_A
  Constant_T_F_86e2c : Constant  Value=T_F
  Constant_V_ref_fef9d : Constant  Value=V_ref
  Constant_f0_4955b : Constant  Value=f0
  Constant_f0_f5ddf : Constant  Value=f0
  Constant_pi_8f988 : Constant  Value=pi
  Constant_pi_ef999 : Constant  Value=pi
  Constant_x_dd_22102 : Constant  Value=x_dd
  Constant_x_dd_9b5d2 : Constant  Value=x_dd
  Constant_x_dd_a4223 : Constant  Value=x_dd
  Constant_x_ddd_3c557 : Constant  Value=x_ddd
  Constant_x_ddd_4a9ac : Constant  Value=x_ddd
  Constant_x_ddd_feab3 : Constant  Value=x_ddd
  Constant_x_l_0c090 : Constant  Value=x_l
  Constant_x_l_13369 : Constant  Value=x_l
  Constant_x_l_9d026 : Constant  Value=x_l
  Constant_x_l_c1452 : Constant  Value=x_l
  Constant_x_l_e028a : Constant  Value=x_l
  Constant_x_l_e4200 : Constant  Value=x_l
  Constant_x_qd_0c5cd : Constant  Value=x_qd
  Constant_x_qd_285d9 : Constant  Value=x_qd
  Constant_x_qd_6c1d7 : Constant  Value=x_qd
  Constant_x_qdd_c2577 : Constant  Value=x_qdd
  Constant_x_qdd_e1cc5 : Constant  Value=x_qdd
  Constant_x_qdd_ed2d6 : Constant  Value=x_qdd
  Divide_55b9e : Product  Inputs=*/
  Divide_5a5da : Product  Inputs=*/
  Divide_97f5d : Product  Inputs=*/
  Divide_a7968 : Product  Inputs=*/
  Divide_c21d6 : Product  Inputs=*/
  Divide_ceadc : Product  Inputs=*/
  Divide_d9ac7 : Product  Inputs=*/
  Divide_dd1f8 : Product  Inputs=*/
  Divide_ecad9 : Product  Inputs=*/
  Divide_feddf : Product  Inputs=*/
  MathFunc_sqrt_17969 : Sqrt
  Power_6d410 : Math  Operator=pow
  Power_bf808 : Math  Operator=pow
  Product_0d32b : Product
  Product_1134f : Product
  Product_2845b : Product
  Product_30bbd : Product
  Product_38feb : Product
  Product_39256 : Product
  Product_40c41 : Product
  Product_61701 : Product
  Product_61a5f : Product
  Product_69bc7 : Product
  Product_6b3a3 : Product
  Product_7006c : Product
  Product_77d96 : Product
  Product_7a789 : Product
  Product_7d8f6 : Product
  Product_9c353 : Product
  Product_9e87b : Product
  Product_a156b : Product
  Product_a446f : Product
  Product_aca70 : Product
  Product_cb62c : Product
  Product_e1797 : Product
  Product_e17a5 : Product
  Subtract_0d251 : Sum  Inputs=+-
  Subtract_4bbba : Sum  Inputs=+-
  Subtract_5b703 : Sum  Inputs=+-
  Subtract_9826f : Sum  Inputs=+-
  Subtract_a59c4 : Sum  Inputs=+-
  Subtract_b979c : Sum  Inputs=+-
  Subtract_d286a : Sum  Inputs=+-
  Subtract_df739 : Sum  Inputs=+-
  Subtract_f726a : Sum  Inputs=+-
  Blockout_d_V_f_SG_D_2_08704 : Outport
  wires:
  Constant_-1_b7bfd/1 -> Product_40c41/1
  Constant_2.0_c254e/1 -> Product_a446f/1
  Constant_-1_34e9f/1 -> Product_1134f/1
  Product_a446f/1 -> Product_a156b/1
  Product_1134f/1 -> Add_970c3/1
  Constant_x_l_e028a/1 -> Product_e17a5/2
  Constant_x_l_9d026/1 -> Product_1134f/2
  State_psi_1d_SG_D_2_6a683/1 -> Product_40c41/2
  Constant_x_l_0c090/1 -> Subtract_b979c/2
  Constant_x_dd_a4223/1 -> Subtract_df739/1
  Product_39256/1 -> Divide_dd1f8/1
  Constant_x_ddd_3c557/1 -> Subtract_df739/2
  Constant_x_qd_285d9/1 -> Add_24c22/2
  Add_970c3/1 -> Product_0d32b/2
  Constant_x_qdd_e1cc5/1 -> Add_970c3/2
  Constant_-1_85a57/1 -> Product_38feb/1
  Constant_x_dd_22102/1 -> Subtract_b979c/1
  Subtract_a59c4/1 -> Add_e1821/1
  Power_bf808/1 -> Add_083c9/1
  Constant_x_l_13369/1 -> Product_38feb/2
  Constant_2.0_f7b41/1 -> Product_aca70/1
  Constant_x_qd_0c5cd/1 -> Subtract_5b703/1
  Constant_pi_ef999/1 -> Product_aca70/2
  Subtract_4bbba/1 -> Product_77d96/2
  Constant_x_qdd_c2577/1 -> Subtract_5b703/2
  State_psi_fd_SG_D_2_5ba3e/1 -> Product_9e87b/1
  Constant_-1_40442/1 -> Product_e17a5/1
  Product_40c41/1 -> Product_e1797/1
  State_w_SG_D_2_1f752/1 -> Product_cb62c/2
  Subtract_df739/1 -> Product_e1797/2
  Constant_x_dd_9b5d2/1 -> Subtract_f726a/1
  State_psi_q_SG_D_2_905ca/1 -> Add_e1821/2
  State_w_SG_D_2_d8cc8/1 -> Product_7d8f6/2
  Subtract_d286a/1 -> Product_9e87b/2
  Constant_x_l_c1452/1 -> Subtract_f726a/2
  Add_77264/1 -> Add_25a22/1
  Constant_x_ddd_4a9ac/1 -> Subtract_d286a/1
  Constant_x_l_e4200/1 -> Subtract_d286a/2
  State_psi_gq_SG_D_2_851e3/1 -> Product_0d32b/1
  Product_38feb/1 -> Add_d7599/1
  Subtract_b979c/1 -> Divide_55b9e/2
  Constant_x_qd_6c1d7/1 -> Add_d7599/2
  Product_7d8f6/1 -> Divide_feddf/1
  State_psi_kq_SG_D_2_52314/1 -> Product_2845b/1
  Subtract_5b703/1 -> Product_2845b/2
  Product_9e87b/1 -> Divide_55b9e/1
  State_V_f_SG_D_2_9fca1/1 -> Subtract_9826f/2
  Product_e17a5/1 -> Add_24c22/1
  Product_e1797/1 -> Divide_ecad9/1
  Divide_a7968/1 -> Subtract_a59c4/1
  Subtract_f726a/1 -> Divide_ecad9/2
  Product_0d32b/1 -> Divide_a7968/1
  Add_d7599/1 -> Divide_a7968/2
  Product_2845b/1 -> Divide_ceadc/1
  Divide_55b9e/1 -> Subtract_4bbba/2
  Constant_f0_f5ddf/1 -> Product_a156b/2
  Add_24c22/1 -> Divide_ceadc/2
  Divide_ecad9/1 -> Add_f0441/1
  State_psi_d_SG_D_2_88c50/1 -> Add_f0441/2
  Divide_ceadc/1 -> Subtract_a59c4/2
  Constant_-1_21c4b/1 -> Product_69bc7/1
  Constant_R_a_04b7e/1 -> Product_69bc7/2
  Constant_f0_4955b/1 -> Product_61701/2
  Add_f0441/1 -> Subtract_4bbba/1
  Product_69bc7/1 -> Product_77d96/1
  Constant_pi_8f988/1 -> Product_a446f/2
  State_psi_q_SG_D_2_113af/1 -> Product_7d8f6/1
  Constant_R_a_90275/1 -> Product_39256/1
  State_E_fd_SG_D_2_a1ee9/1 -> Product_9c353/2
  Add_e1821/1 -> Product_39256/2
  State_psi_d_SG_D_2_b6804/1 -> Product_cb62c/1
  Product_aca70/1 -> Product_61701/1
  Product_77d96/1 -> Divide_c21d6/1
  Constant_x_ddd_feab3/1 -> Divide_c21d6/2
  Product_a156b/1 -> Divide_feddf/2
  Constant_x_qdd_ed2d6/1 -> Divide_dd1f8/2
  Product_cb62c/1 -> Divide_5a5da/1
  Product_61701/1 -> Divide_5a5da/2
  Divide_c21d6/1 -> Add_b86ea/1
  Divide_feddf/1 -> Add_b86ea/2
  Divide_dd1f8/1 -> Add_aac42/1
  Divide_5a5da/1 -> Add_aac42/2
  Constant_-1_ac8df/1 -> Product_9c353/1
  Add_b86ea/1 -> Power_bf808/1
  Constant_2.0_f026f/1 -> Power_bf808/2
  Add_aac42/1 -> Power_6d410/1
  Constant_2.0_c78cc/1 -> Power_6d410/2
  Product_9c353/1 -> Product_7a789/1
  Constant_K_A_15ed7/1 -> Product_7a789/2
  Constant_K_s_f6b89/1 -> Product_7006c/1
  State_Px_3_SG_D_2_37027/1 -> Product_7006c/2
  Power_6d410/1 -> Add_083c9/2
  Product_7a789/1 -> Product_61a5f/1
  Constant_K_F_50d73/1 -> Product_61a5f/2
  Product_7006c/1 -> Add_bee69/1
  Constant_V_ref_fef9d/1 -> Add_bee69/2
  Add_083c9/1 -> MathFunc_sqrt_17969/1
  Product_61a5f/1 -> Divide_97f5d/1
  Constant_T_F_86e2c/1 -> Divide_97f5d/2
  Constant_K_A_a5957/1 -> Product_6b3a3/1
  State_R_f_SG_D_2_2b1aa/1 -> Product_6b3a3/2
  Add_bee69/1 -> Subtract_0d251/1
  MathFunc_sqrt_17969/1 -> Subtract_0d251/2
  Divide_97f5d/1 -> Add_77264/1
  Product_6b3a3/1 -> Add_77264/2
  Constant_K_A_822bf/1 -> Product_30bbd/1
  Subtract_0d251/1 -> Product_30bbd/2
  Product_30bbd/1 -> Add_25a22/2
  Add_25a22/1 -> Subtract_9826f/1
  Subtract_9826f/1 -> Divide_d9ac7/1
  Constant_T_A_713ce/1 -> Divide_d9ac7/2
  Divide_d9ac7/1 -> Blockout_d_V_f_SG_D_2_08704/1

== system case4/SG_D_2/d_psi_1d_SG_D_2_block ==
  note: d_psi_1d_SG_D_2 in case4
      | $-\frac{\psi _{\mathrm{1d},\mathrm{SG},D,2}-\psi _{\mathrm{fd},\mathrm{SG},D,2}+\frac{\left(x_{\mathrm{dd}}-x_{l}\right)\,\left(\frac{\psi _{\mathrm{1d},\mathrm{SG},D,2}\,\left(x_{\mathrm{dd}}-x_{\mathrm{ddd}}\right)}{x_{\mathrm{dd}}-x_{l}}-\psi _{d,\mathrm{SG},D,2}+\frac{\psi _{\mathrm{fd},\mathrm{SG},D,2}\,\left(x_{\mathrm{ddd}}-x_{l}\right)}{x_{\mathrm{dd}}-x_{l}}\right)}{x_{\mathrm{ddd}}}}{T_{\mathrm{ddd}}}$
      | Automatically generated on 2025-10-31 19:05:24 .
  State_psi_1d_SG_D_2_89b76 : Inport
  State_psi_fd_SG_D_2_d4a3d : Inport  Port=2
  State_psi_1d_SG_D_2_48a12 : Inport  Port=3
  State_psi_d_SG_D_2_8f652 : Inport  Port=4
  State_psi_fd_SG_D_2_2139b : Inport  Port=5
  Add_1510f : Sum
  Add_a5bd4 : Sum
  Add_b8afc : Sum
  Constant_-1_0dde9 : Constant  Value=-1
  Constant_-1_1b067 : Constant  Value=-1
  Constant_T_ddd_e79da : Constant  Value=T_ddd
  Constant_x_dd_198e5 : Constant  Value=x_dd
  Constant_x_dd_5df1e : Constant  Value=x_dd
  Constant_x_dd_66e28 : Constant  Value=x_dd
  Constant_x_dd_70158 : Constant  Value=x_dd
  Constant_x_ddd_01cbb : Constant  Value=x_ddd
  Constant_x_ddd_77dde : Constant  Value=x_ddd
  Constant_x_ddd_9cdc7 : Constant  Value=x_ddd
  Constant_x_l_538a1 : Constant  Value=x_l
  Constant_x_l_6934b : Constant  Value=x_l
  Constant_x_l_a667e : Constant  Value=x_l
  Constant_x_l_b9a1d : Constant  Value=x_l
  Divide_007b4 : Product  Inputs=*/
  Divide_3f051 : Product  Inputs=*/
  Divide_87d5a : Product  Inputs=*/
  Divide_a0e47 : Product  Inputs=*/
  Product_5abd0 : Product
  Product_7361e : Product
  Product_8c34d : Product
  Product_aed7a : Product
  Product_f941f : Product
  Subtract_059f6 : Sum  Inputs=+-
  Subtract_40d59 : Sum  Inputs=+-
  Subtract_5b3fb : Sum  Inputs=+-
  Subtract_8be25 : Sum  Inputs=+-
  Subtract_9975a : Sum  Inputs=+-
  Subtract_f53c8 : Sum  Inputs=+-
  Blockout_d_psi_1d_SG_D_2_0e78a : Outport
  wires:
  Subtract_9975a/1 -> Product_8c34d/2
  Constant_x_l_a667e/1 -> Subtract_059f6/2
  Divide_87d5a/1 -> Add_a5bd4/2
  Subtract_5b3fb/1 -> Product_f941f/2
  Constant_-1_0dde9/1 -> Product_7361e/1
  Constant_x_dd_66e28/1 -> Subtract_f53c8/1
  Divide_007b4/1 -> Blockout_d_psi_1d_SG_D_2_0e78a/1
  State_psi_fd_SG_D_2_d4a3d/1 -> Add_b8afc/2
  State_psi_1d_SG_D_2_48a12/1 -> Product_7361e/2
  Divide_a0e47/1 -> Subtract_5b3fb/2
  Constant_x_ddd_77dde/1 -> Subtract_f53c8/2
  State_psi_1d_SG_D_2_89b76/1 -> Product_5abd0/2
  Product_7361e/1 -> Product_aed7a/1
  Subtract_f53c8/1 -> Product_aed7a/2
  Constant_x_dd_70158/1 -> Subtract_059f6/1
  Constant_x_ddd_9cdc7/1 -> Subtract_9975a/1
  Constant_x_l_6934b/1 -> Subtract_9975a/2
  Product_aed7a/1 -> Divide_3f051/1
  Subtract_059f6/1 -> Divide_3f051/2
  State_psi_fd_SG_D_2_2139b/1 -> Product_8c34d/1
  Constant_x_dd_198e5/1 -> Subtract_8be25/1
  Constant_x_l_538a1/1 -> Subtract_40d59/2
  Constant_x_l_b9a1d/1 -> Subtract_8be25/2
  Constant_x_ddd_01cbb/1 -> Divide_87d5a/2
  Divide_3f051/1 -> Add_1510f/1
  State_psi_d_SG_D_2_8f652/1 -> Add_1510f/2
  Product_8c34d/1 -> Divide_a0e47/1
  Subtract_8be25/1 -> Divide_a0e47/2
  Constant_x_dd_5df1e/1 -> Subtract_40d59/1
  Add_1510f/1 -> Subtract_5b3fb/1
  Constant_-1_1b067/1 -> Product_5abd0/1
  Subtract_40d59/1 -> Product_f941f/1
  Product_5abd0/1 -> Add_b8afc/1
  Product_f941f/1 -> Divide_87d5a/1
  Add_b8afc/1 -> Add_a5bd4/1
  Add_a5bd4/1 -> Divide_007b4/1
  Constant_T_ddd_e79da/1 -> Divide_007b4/2
